simulink model "GFMGFL_9bus_v1"  (R2024b)
settings: Solver=FixedStepAuto  StartTime=0  StopTime=5  FixedStep=Ts  RelTol=1e-3
values from neighbouring files (symbols this model uses):
  ApparatusDiscreDamping =     [WSCC_9Bus_Workspace.mat]
  ApparatusPara =     [WSCC_9Bus_Workspace.mat]
  ApparatusPowerFlow =     [WSCC_9Bus_Workspace.mat]
  ApparatusType =     [WSCC_9Bus_Workspace.mat]
  OtherInputs =     [WSCC_9Bus_Workspace.mat]
  Ts = 3.33333333333e-05    [WSCC_9Bus_Workspace.mat]
  Wbase = 376.991118431    [WSCC_9Bus_Workspace.mat]
  x_e =     [WSCC_9Bus_Workspace.mat]
  Ybase = 1    [WSCC_9Bus_Workspace.mat]
  Zbase = 1    [WSCC_9Bus_Workspace.mat]
libraries: SimplusGT x12, spsGroundLib x9, spsThreePhaseSeriesRLCBranchLib x9, spsThreePhaseParallelRLCBranchLib x6, sps_lib x1
settings Model: Creator=皮蛋蛋挞  LastModifiedBy=皮蛋蛋挞

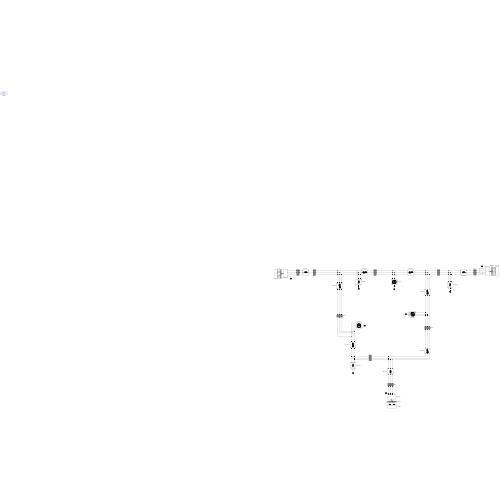
[thumbnail: Simulink's stored preview of the top-level diagram]
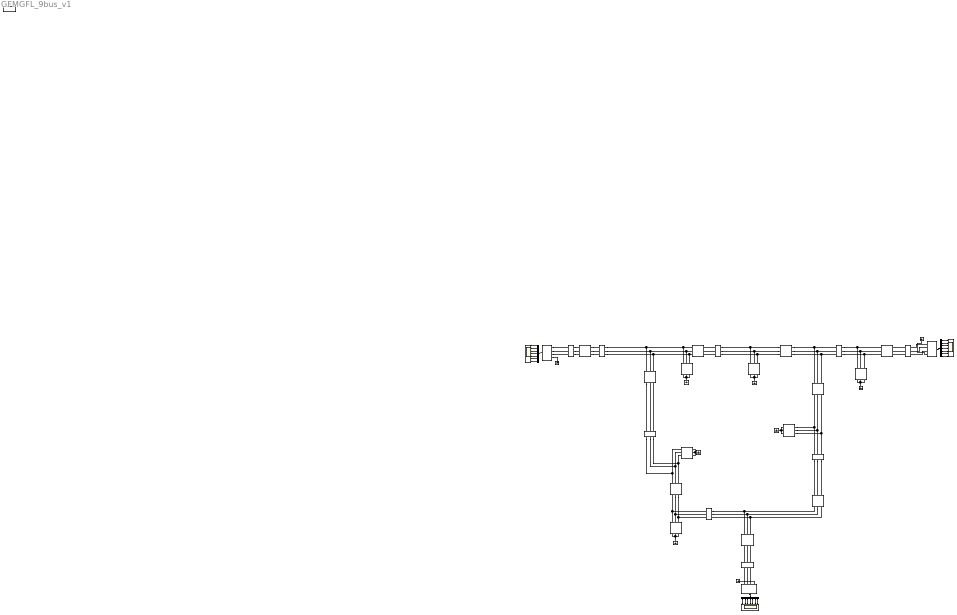
== system GFMGFL_9bus_v1 ==
  B-GND{4,7,9,11,13,15} (6 alike) : spsGroundLib/Ground  LConnTagsString=a
  Branch1-4 : spsThreePhaseSeriesRLCBranchLib/Three-Phase Series RLC Branch  LConnTagsString=A|B|C  RConnTagsString=A|B|C  BranchType=L  Resistance=(0)*Zbase  Inductance=(0.0576)*Zbase/Wbase  Capacitance=1e-6  Measurements=None
  Branch2-7 : spsThreePhaseSeriesRLCBranchLib/Three-Phase Series RLC Branch  LConnTagsString=A|B|C  RConnTagsString=A|B|C  BranchType=L  Resistance=(0)*Zbase  Inductance=(0.0625)*Zbase/Wbase  Capacitance=1e-6  Measurements=None
  Branch3-9 : spsThreePhaseSeriesRLCBranchLib/Three-Phase Series RLC Branch  LConnTagsString=A|B|C  RConnTagsString=A|B|C  BranchType=L  Resistance=(0)*Zbase  Inductance=(0.0586)*Zbase/Wbase  Capacitance=1e-6  Measurements=None
  Branch4-4 : spsThreePhaseParallelRLCBranchLib/Three-Phase Parallel RLC Branch  LConnTagsString=A|B|C  RConnTagsString=A|B|C  BranchType=C  Resistance=(Inf)*Zbase  Inductance=(Inf)*Zbase/Wbase  Capacitance=(0.167)*Ybase/Wbase  Measurements=None
  Branch4-5 : spsThreePhaseSeriesRLCBranchLib/Three-Phase Series RLC Branch  LConnTagsString=A|B|C  RConnTagsString=A|B|C  BranchType=RL  Resistance=(0.01)*Zbase  Inductance=(0.085)*Zbase/Wbase  Capacitance=1e-6  Measurements=None
  Branch4-6 : spsThreePhaseSeriesRLCBranchLib/Three-Phase Series RLC Branch  LConnTagsString=A|B|C  RConnTagsString=A|B|C  BranchType=RL  Resistance=(0.017)*Zbase  Inductance=(0.092)*Zbase/Wbase  Capacitance=1e-6  Measurements=None
  Branch5-5 : spsThreePhaseParallelRLCBranchLib/Three-Phase Parallel RLC Branch  LConnTagsString=A|B|C  RConnTagsString=A|B|C  BranchType=RLC  Resistance=(0.79302)*Zbase  Inductance=(1.9826)*Zbase/Wbase  Capacitance=(0.241)*Ybase/Wbase  Measurements=None
  Branch5-7 : spsThreePhaseSeriesRLCBranchLib/Three-Phase Series RLC Branch  LConnTagsString=A|B|C  RConnTagsString=A|B|C  BranchType=RL  Resistance=(0.032)*Zbase  Inductance=(0.161)*Zbase/Wbase  Capacitance=1e-6  Measurements=None
  Branch6-6 : spsThreePhaseParallelRLCBranchLib/Three-Phase Parallel RLC Branch  LConnTagsString=A|B|C  RConnTagsString=A|B|C  BranchType=RLC  Resistance=(1.1394)*Zbase  Inductance=(3.4182)*Zbase/Wbase  Capacitance=(0.258)*Ybase/Wbase  Measurements=None
  Branch6-9 : spsThreePhaseSeriesRLCBranchLib/Three-Phase Series RLC Branch  LConnTagsString=A|B|C  RConnTagsString=A|B|C  BranchType=RL  Resistance=(0.039)*Zbase  Inductance=(0.17)*Zbase/Wbase  Capacitance=1e-6  Measurements=None
  Branch7-7 : spsThreePhaseParallelRLCBranchLib/Three-Phase Parallel RLC Branch  LConnTagsString=A|B|C  RConnTagsString=A|B|C  BranchType=C  Resistance=(Inf)*Zbase  Inductance=(Inf)*Zbase/Wbase  Capacitance=(0.2275)*Ybase/Wbase  Measurements=None
  Branch7-8 : spsThreePhaseSeriesRLCBranchLib/Three-Phase Series RLC Branch  LConnTagsString=A|B|C  RConnTagsString=A|B|C  BranchType=RL  Resistance=(0.0085)*Zbase  Inductance=(0.072)*Zbase/Wbase  Capacitance=1e-6  Measurements=None
  Branch8-8 : spsThreePhaseParallelRLCBranchLib/Three-Phase Parallel RLC Branch  LConnTagsString=A|B|C  RConnTagsString=A|B|C  BranchType=RLC  Resistance=(1.032)*Zbase  Inductance=(2.9486)*Zbase/Wbase  Capacitance=(0.179)*Ybase/Wbase  Measurements=None
  Branch8-9 : spsThreePhaseSeriesRLCBranchLib/Three-Phase Series RLC Branch  LConnTagsString=A|B|C  RConnTagsString=A|B|C  BranchType=RL  Resistance=(0.0119)*Zbase  Inductance=(0.1008)*Zbase/Wbase  Capacitance=1e-6  Measurements=None
  Branch9-9 : spsThreePhaseParallelRLCBranchLib/Three-Phase Parallel RLC Branch  LConnTagsString=A|B|C  RConnTagsString=A|B|C  BranchType=C  Resistance=(Inf)*Zbase  Inductance=(Inf)*Zbase/Wbase  Capacitance=(0.2835)*Ybase/Wbase  Measurements=None
  Bus{1..9} (9 alike) : SimplusGT/Three-Phase Bus  Vbase=1  Sbase=1
  D-GND1 : spsGroundLib/Ground  LConnTagsString=a
  D-GND2 : spsGroundLib/Ground  LConnTagsString=a
  D-GND3 : spsGroundLib/Ground  LConnTagsString=a
  D-Scope1 : Scope  NumInputPorts=7
  D-Scope2 : Scope  NumInputPorts=7
  D-Scope3 : Scope  NumInputPorts=7
  DS-Bus1 : BusSelector  OutputSignals=v_dq,i_dq,v_abc,i_abc,w,theta,pq
  DS-Bus2 : BusSelector  OutputSignals=v_dq,i_dq,v_abc,i_abc,w,theta,pq
  DS-Bus3 : BusSelector  OutputSignals=v_dq,i_dq,v_abc,i_abc,w,theta,pq
  VSI-Droop1 : SimplusGT/Grid-Forming Voltage-Source Inverter (dq-Frame System Object)  Ts=Ts  Sbase=Sbase  Vbase=Vbase  Wbase=Wbase  ApparatusType=ApparatusType{1}  ApparatusPara=ApparatusPara{1}  PowerFlow=ApparatusPowerFlow{1}  x0=x_e{1}  OtherInputs=OtherInputs{1}  DiscreMethod=Hybrid Trapezoidal  EnableInsideModification=off  DiscreDampingFlag=on  DiscreDampingValue=ApparatusDiscreDamping{1}  LinearizationTimes=1  DirectFeedthrough=off
  VSI-Droop3 : SimplusGT/Grid-Forming Voltage-Source Inverter (dq-Frame System Object)  Ts=Ts  Sbase=Sbase  Vbase=Vbase  Wbase=Wbase  ApparatusType=ApparatusType{3}  ApparatusPara=ApparatusPara{3}  PowerFlow=ApparatusPowerFlow{3}  x0=x_e{3}  OtherInputs=OtherInputs{3}  DiscreMethod=Hybrid Trapezoidal  EnableInsideModification=off  DiscreDampingFlag=on  DiscreDampingValue=ApparatusDiscreDamping{3}  LinearizationTimes=1  DirectFeedthrough=off
  VSI-PLL2 : SimplusGT/Grid-Following Voltage-Source Inverter (dq-Frame System Object)  Ts=Ts  Sbase=Sbase  Vbase=Vbase  Wbase=Wbase  ApparatusType=ApparatusType{2}  ApparatusPara=ApparatusPara{2}  PowerFlow=ApparatusPowerFlow{2}  x0=x_e{2}  OtherInputs=OtherInputs{2}  DiscreMethod=Hybrid Trapezoidal  EnableInsideModification=off  DiscreDampingFlag=on  DiscreDampingValue=ApparatusDiscreDamping{2}  LinearizationTimes=1  DirectFeedthrough=off
  powergui : sps_lib/powergui  Priority=1  SimulationMode=Discrete  SampleTime=Ts  frequency=60  Iterations=50  frequencyindice=0  Pbase=100e6  ErrMax=1e-4  UnitsV=kV  UnitsW=MW  buscounter=0  FunctionMessages=off  echomessages=off  EnableUseOfTLC=off  CurrentSourceSwitches=off  DisableSnubberDevices=off  DisableRonSwitches=off  DisableVfSwitches=off  DisplayEquations=off  AutomaticDiscreteSolvers=off  SolverType=Tustin/Backward Euler (TBE)  Interpol=off  ExternalGateDelay=off  methode=off  Ts=100  x0status=blocks  SPID=on  SwTol=0  HookPort=off  NonlinearTolerance=1e-4  nMaxIteration=100  ContinueOnMaxIteration=off  RestoreLinks=warning  ResistiveCurrentMeasurement=off  Frange=[0:2:500]  Ylog=off  Xlog=on  ShowGrid=off  save=off  variable=ZData  structure=0  ZoomFFT=off  StartTime=0.0  cycles=1  DisplayStyle=1  fundamental=60  FreqAxis=off  MaxFrequency=1000  frequencyindicesteady=1  RmsSteady=1  display=off
  wires:
  VSI-Droop1/1 -> DS-Bus1/1
  DS-Bus1/1 -> D-Scope1/1  "<v_dq>"
  DS-Bus1/2 -> D-Scope1/2  "<i_dq>"
  DS-Bus1/3 -> D-Scope1/3  "<v_abc>"
  DS-Bus1/4 -> D-Scope1/4  "<i_abc>"
  DS-Bus1/5 -> D-Scope1/5  "<w>"
  DS-Bus1/6 -> D-Scope1/6  "<theta>"
  DS-Bus1/7 -> D-Scope1/7  "<pq>"
  VSI-PLL2/1 -> DS-Bus2/1
  DS-Bus2/1 -> D-Scope2/1  "<v_dq>"
  DS-Bus2/2 -> D-Scope2/2  "<i_dq>"
  DS-Bus2/3 -> D-Scope2/3  "<v_abc>"
  DS-Bus2/4 -> D-Scope2/4  "<i_abc>"
  DS-Bus2/5 -> D-Scope2/5  "<w>"
  DS-Bus2/6 -> D-Scope2/6  "<theta>"
  DS-Bus2/7 -> D-Scope2/7  "<pq>"
  VSI-Droop3/1 -> DS-Bus3/1
  DS-Bus3/1 -> D-Scope3/1  "<v_dq>"
  DS-Bus3/2 -> D-Scope3/2  "<i_dq>"
  DS-Bus3/3 -> D-Scope3/3  "<v_abc>"
  DS-Bus3/4 -> D-Scope3/4  "<i_abc>"
  DS-Bus3/5 -> D-Scope3/5  "<w>"
  DS-Bus3/6 -> D-Scope3/6  "<theta>"
  DS-Bus3/7 -> D-Scope3/7  "<pq>"
  connections:
  VSI-Droop1/LConn4 -- D-GND1/LConn1
  VSI-PLL2/LConn4 -- D-GND2/LConn1
  VSI-Droop3/LConn4 -- D-GND3/LConn1
  Branch4-4/RConn2 -- Branch4-4/RConn3 -- B-GND4/LConn1 -- Branch4-4/RConn1
  Branch5-5/RConn2 -- Branch5-5/RConn3 -- Branch5-5/RConn1 -- B-GND7/LConn1
  Branch6-6/RConn2 -- Branch6-6/RConn1 -- B-GND9/LConn1 -- Branch6-6/RConn3
  Branch7-7/RConn2 -- B-GND11/LConn1 -- Branch7-7/RConn1 -- Branch7-7/RConn3
  Branch8-8/RConn1 -- Branch8-8/RConn2 -- Branch8-8/RConn3 -- B-GND13/LConn1
  B-GND15/LConn1 -- Branch9-9/RConn3 -- Branch9-9/RConn2 -- Branch9-9/RConn1
  Branch4-4/LConn1 -- Bus4/RConn1 -- Branch4-5/LConn1
  Branch4-6/LConn2 -- Branch1-4/RConn2 -- Bus4/LConn2
  Branch4-6/LConn3 -- Branch1-4/RConn3 -- Bus4/LConn3
  Bus1/RConn1 -- Branch1-4/LConn1
  Bus1/RConn2 -- Branch1-4/LConn2
  Bus1/RConn3 -- Branch1-4/LConn3
  Bus7/RConn1 -- Branch5-7/RConn1 -- Branch7-8/LConn1 -- Branch7-7/LConn1
  Bus7/RConn2 -- Branch5-7/RConn2 -- Branch7-8/LConn2 -- Branch7-7/LConn2
  Bus7/RConn3 -- Branch5-7/RConn3 -- Branch7-8/LConn3 -- Branch7-7/LConn3
  Bus2/RConn1 -- Branch2-7/LConn1
  Bus2/RConn2 -- Branch2-7/LConn2
  Bus2/RConn3 -- Branch2-7/LConn3
  Bus3/RConn1 -- Branch3-9/LConn1
  Bus3/RConn2 -- Branch3-9/LConn2
  Bus3/RConn3 -- Branch3-9/LConn3
  Branch5-5/LConn1 -- Bus5/LConn1 -- Branch4-5/RConn1
  Branch5-5/LConn2 -- Bus5/LConn2 -- Branch4-5/RConn2
  Bus6/LConn1 -- Branch4-6/RConn1
  Bus6/LConn2 -- Branch4-6/RConn2
  Bus6/LConn3 -- Branch4-6/RConn3
  Branch8-9/LConn1 -- Branch8-8/LConn1 -- Bus8/RConn1
  Branch8-9/LConn2 -- Branch8-8/LConn2 -- Bus8/RConn2
  Branch8-9/LConn3 -- Branch8-8/LConn3 -- Bus8/RConn3
  VSI-Droop1/LConn1 -- Bus1/LConn1
  VSI-Droop1/LConn2 -- Bus1/LConn2
  VSI-Droop1/LConn3 -- Bus1/LConn3
  VSI-PLL2/LConn1 -- Bus2/LConn1
  VSI-PLL2/LConn2 -- Bus2/LConn2
  VSI-PLL2/LConn3 -- Bus2/LConn3
  VSI-Droop3/LConn1 -- Bus3/LConn1
  VSI-Droop3/LConn2 -- Bus3/LConn2
  VSI-Droop3/LConn3 -- Bus3/LConn3
  Branch2-7/RConn3 -- Bus7/LConn3
  Branch2-7/RConn2 -- Bus7/LConn2
  Branch2-7/RConn1 -- Bus7/LConn1
  Bus8/LConn1 -- Branch7-8/RConn1
  Bus8/LConn2 -- Branch7-8/RConn2
  Bus8/LConn3 -- Branch7-8/RConn3
  Branch8-9/RConn1 -- Branch6-9/RConn1 -- Bus9/LConn1
  Branch8-9/RConn2 -- Branch6-9/RConn2 -- Bus9/LConn2
  Branch8-9/RConn3 -- Branch6-9/RConn3 -- Bus9/LConn3
  Bus9/RConn1 -- Branch9-9/LConn1 -- Branch3-9/RConn1
  Bus9/RConn2 -- Branch9-9/LConn2 -- Branch3-9/RConn2
  Bus9/RConn3 -- Branch9-9/LConn3 -- Branch3-9/RConn3
  Branch5-7/LConn1 -- Bus5/RConn1
  Bus5/RConn2 -- Branch5-7/LConn2
  Bus5/RConn3 -- Branch5-7/LConn3
  Branch5-5/LConn3 -- Bus5/LConn3 -- Branch4-5/RConn3
  Branch4-5/LConn2 -- Bus4/RConn2 -- Branch4-4/LConn2
  Branch4-6/LConn1 -- Branch1-4/RConn1 -- Bus4/LConn1
  Bus4/RConn3 -- Branch4-5/LConn3 -- Branch4-4/LConn3
  Bus6/RConn1 -- Branch6-6/LConn1 -- Branch6-9/LConn1
  Bus6/RConn2 -- Branch6-6/LConn2 -- Branch6-9/LConn2
  Bus6/RConn3 -- Branch6-6/LConn3 -- Branch6-9/LConn3
